simulink model "magnetometer"  (R2015a)
settings: Solver=ode45  StartTime=0.0  StopTime=10  RelTol=1e-3
undefined symbols (not defined in the file): magMax, magNoise, magOffset
libraries: simulink x1
settings Model: Creator=johnz  LastModifiedBy=johnz

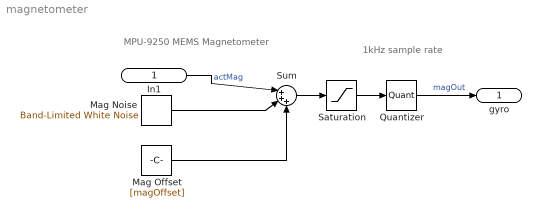
== system magnetometer ==
  note: MPU-9250 MEMS Magnetometer
  note: 1kHz sample rate
  In1 : Inport
  Mag Noise : simulink/Sources/Band-Limited White Noise  Cov=[magNoise]  Ts=1/1000  seed=[10]
  Mag Offset : Constant  Value=[magOffset]
  Quantizer : Quantizer  QuantizationInterval=magSensitivity
  Saturation : Saturate  UpperLimit=magMax  LowerLimit=-magMax
  Sum : Sum  Inputs=|+++
  gyro : Outport  OutDataTypeStr=double  PortDimensions=1
  wires:
  In1/1 -> Sum/1  "actMag"
  Sum/1 -> Saturation/1
  Saturation/1 -> Quantizer/1
  Mag Offset/1 -> Sum/3
  Quantizer/1 -> gyro/1  "magOut"
  Mag Noise/1 -> Sum/2
